simulink model "simulink_1a_S"  (R2020b)
settings: Solver=VariableStepAuto  StartTime=0.0  StopTime=10.0  MaxStep=1e-4  RelTol=1e-3
values from neighbouring files (symbols this model uses):
  A = [0,1; (aa*sqrt(2)*Fv)/(4*Id), -beta/Id]    [Progetto_1a_gruppoS.m]
  aa = 0.3    [Progetto_1a_gruppoS.m]
  B = [0;aa/Id]    [Progetto_1a_gruppoS.m]
  beta = 0.3    [Progetto_1a_gruppoS.m]
  C = [1,0]    [Progetto_1a_gruppoS.m]
  den_r = d_r{1}    [Progetto_1a_gruppoS.m]
  Fv = -8.7    [Progetto_1a_gruppoS.m]
  Id = 0.5    [Progetto_1a_gruppoS.m]
  num_r = n_r{1}    [Progetto_1a_gruppoS.m]
  omega_n = 12000    [Progetto_1a_gruppoS.m]
  u_e = (-sqrt(2)*Fv)/4    [Progetto_1a_gruppoS.m]
  W = -pi/4    (= -0.785398163397)    [Progetto_1a_gruppoS.m]
  x0 = [pi/4;0]    [Progetto_1a_gruppoS.m]
  y_e = pi/4    (= 0.785398163397)    [Progetto_1a_gruppoS.m]
settings Model: Creator=spiri  LastModifiedBy=jacopo

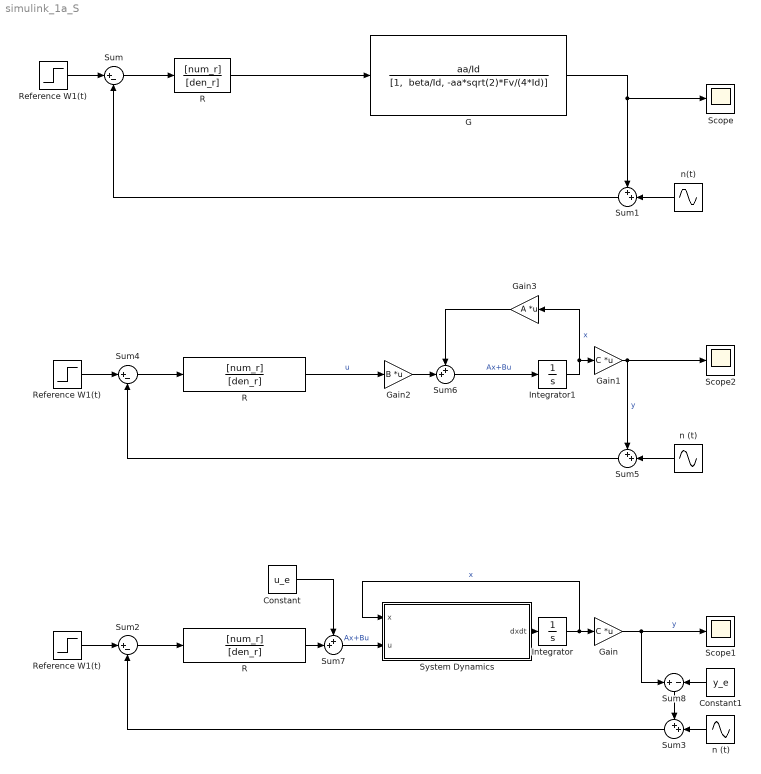
== system simulink_1a_S ==
  Constant : Constant  Value=u_e
  Constant1 : Constant  Value=y_e
  G : TransferFcn  Numerator=aa/Id  Denominator="[1,  beta/Id, -aa*sqrt(2)*Fv/(4*Id)]"
  Gain : Gain  Gain=C  Multiplication=Matrix(K*u)
  Gain1 : Gain  Gain=C  Multiplication=Matrix(K*u)
  Gain2 : Gain  Gain=B  Multiplication=Matrix(K*u)
  Gain3 : Gain  Gain=A  Multiplication=Matrix(K*u)
  Integrator : Integrator  InitialCondition=x0
  Integrator1 : Integrator  InitialCondition=x0
  R : TransferFcn  Numerator=[num_r]  Denominator=[den_r]
  "R " : TransferFcn  Numerator=[num_r]  Denominator=[den_r]
  "R " : TransferFcn  Numerator=[num_r]  Denominator=[den_r]
  Reference W1(t) : Step  After=W  SampleTime=0
  "Reference W1(t) " : Step  Time=0  After=W  SampleTime=0
  "Reference W1(t) " : Step  After=W  SampleTime=0
  Scope : Scope
  Scope1 : Scope
  Scope2 : Scope
  Sum : Sum  Inputs=|+-
  Sum{1,3,5..7} (5 alike) : Sum  Inputs=++|
  Sum2 : Sum  Inputs=|+-
  Sum4 : Sum  Inputs=|+-
  Sum8 : Sum  Inputs=+-
  System Dynamics : MATLAB Function  TreatAsAtomicUnit=on
  n (t) : Sin  Amplitude=0.01  Frequency=omega_n  SampleTime=0
  "n (t) " : Sin  Amplitude=0.01  Frequency=omega_n  SampleTime=0
  n(t) : Sin  Amplitude=0.01  Frequency=omega_n  SampleTime=0
  wires:
  n(t)/1 -> Sum1/2
  Sum1/1 -> Sum/2
  Reference W1(t)/1 -> Sum/1
  G/1 -> Scope/1, Sum1/1
  Sum/1 -> R/1
  R/1 -> G/1
  "R "/1 -> Sum7/2
  Sum2/1 -> "R "/1
  "Reference W1(t) "/1 -> Sum2/1
  Sum3/1 -> Sum2/2
  n (t)/1 -> Sum3/2
  System Dynamics/1(dxdt) -> Integrator/1
  Integrator/1 -> System Dynamics/1(x), Gain/1  "x"
  Gain/1 -> Sum8/1, Scope1/1  "y"
  Gain1/1 -> Sum5/1, Scope2/1  "y"
  Integrator1/1 -> Gain1/1, Gain3/1  "x"
  Sum6/1 -> Integrator1/1  "Ax+Bu"
  "n (t) "/1 -> Sum5/2
  Sum5/1 -> Sum4/2
  "Reference W1(t) "/1 -> Sum4/1
  Sum4/1 -> "R "/1
  "R "/1 -> Gain2/1  "u"
  Gain2/1 -> Sum6/2
  Gain3/1 -> Sum6/1
  Sum7/1 -> System Dynamics/2(u)  "Ax+Bu"
  Constant/1 -> Sum7/1
  Constant1/1 -> Sum8/2
  Sum8/1 -> Sum3/1

== matlab function simulink_1a_S/System Dynamics ==
  data: x input; u input; dxdt output
function dxdt = systemDynamics(x,u)

Id=0.5;     %[kg*m^2] Momento di Inerzia del drone rispetto all'asse di rotazione
beta=0.3;   %[] Coefficiente di attrito dinamico dovuto all'aria
aa=0.3;     %[m] Distanza dai punti di applicazione delle forze al baricentro
Fv=-8.7;    %[N] Forza del vento

%%System dynamics
% dot{x_1}=x_2
% dot{x_2}mm=(-beta*x_2+aa/2*sin(x_1)*Fv+aa*u_1)/Id
% y=x_1


dx1dt=x(2);
dx2dt= ( -beta* x(2) + aa/2 *sin( x(1) )*Fv+aa* u(1) ) /Id
%dxdt = [dx1dt; dx2dt; dx3dt;...;dxndt];
dxdt = [dx1dt; dx2dt;];
